simulink library "ddm"  (R2021b)
settings: Solver=VariableStepAuto  StartTime=0.0  StopTime=10.0  RelTol=1e-3
undefined symbols (not defined in the file): ADDM_FrTMTqDev_X_Nm, ADDM_RrTMTqDev_X_Nm, ENUM_ADASACCSTA_ERROR, ENUM_ADASACCSTA_OFF, ENUM_ADASACCSTA_STANDBY, ENUM_ALLOWMOV_ALLOWREADY, ENUM_APS, ENUM_BRKSTA_ERROR, ENUM_BRKSTA_OFF, ENUM_BRKSTA_ON, ENUM_BRKSW_INVALID, ENUM_BRKSW_OFF, ENUM_BRKSW_ON, ENUM_CHGPREACTERRSTA_OBCPRE, ENUM_DCDCFAULTSTA_ANYFAULTLV1, ENUM_DCDCFAULTSTA_ANYFAULTLV2, ENUM_DRIVETRAIN_AWD, ENUM_DRIVETRAIN_FWD, ENUM_DRIVETRAIN_RWD, ENUM_EDUDRTSTA_NORMAL, ENUM_EPBERROR_FAILED, ENUM_EPBSTA_APPLIED, ENUM_EPBSTA_RELEASED, ENUM_ESCAPSSta_APSUNAVAILABLE, ENUM_GEARACTUALPOSN_INVALID, ENUM_GEARACTUALPOSN_P, ENUM_HVBATTREADYPRE_READY, ENUM_HWRESETSTA_HWRESETING, ENUM_MCUWARN_LV0, ENUM_MCUWARN_LV1, ENUM_MCUWARN_LV2, ENUM_MCUWARN_LV3, ENUM_MCUWARN_NOERROR, ENUM_OBCFAULTSTA_ANYFAULT, ENUM_PAS_R2F2, ENUM_PDFAULT_BATTPDFAIL, ENUM_PDFAULT_DCDCDISABLE, ENUM_PDFAULT_MCUDISABLE, ENUM_PDFAULT_MCUDISCHRG, ENUM_POWERSTA_OFF, ENUM_POWERSTA_ON, ENUM_POWERSTA_READY, ENUM_POWERSTA_STANDBY, ENUM_PRESSINDI_LOW, ENUM_PUFAULT_BATTUPFAIL, ENUM_PUFAULT_DCDCENABLEFAIL, ENUM_PUFAULT_PRECHRGCHKFAIL, ENUM_PUFAULT_SAFETYCHKFAIL, ENUM_PWRSTASW_OFF, ENUM_PWRSTASW_OFFA, ENUM_PWRSTASW_OFFCHVCHRG, ENUM_PWRSTASW_OFFCLVCHRG, ENUM_PWRSTASW_ON, ENUM_PWRSTASW_ONHVCHRG, ENUM_PWRSTASW_READY, ENUM_PWRSTASW_STANDBY, ENUM_RAPSErrWarnSta_NORMAL, ENUM_RAPSErrWarnSta_RAPSERRLV1, ENUM_SHIFTCOMMAND_P, ENUM_SHIFTERERRSTA_PBUTTONFAILURE ... (+471)
libraries: hcu_lib x540, simulink x3
(part 8 of 26)

== system ddm/DDM/DDM/APM/Subsystem5 ==
  USSSta_flg : Inport
  VPMM_SysPwrSta_enum : Inport  Port=2
  VAPM_SNSRLayout_enum : Inport  Port=3
  Constant1 : Constant  Value=ENUM_PWRSTASW_READY
  Constant17 : Constant  Value=ENUM_PWRSTASW_READY
  Constant2 : Constant  Value=ENUM_PWRSTASW_ON
  Constant25 : Constant  Value=FALSE
  Constant3 : Constant  Value=ENUM_PWRSTASW_ON
  Constant4 : Constant  Value=ENUM_APS
  Constant5 : Constant  Value=ENUM_PAS_R2F2
  Equal{1..6} (6 alike) : RelationalOperator  Operator===  OutDataTypeStr=boolean  RndMeth=Simplest
  Logical Operator1 : Logic  Operator=NOT  AllPortsSameDT=off  OutDataTypeStr=boolean
  Logical Operator13 : Logic  Operator=OR  AllPortsSameDT=off  OutDataTypeStr=boolean
  Logical Operator2 : Logic  AllPortsSameDT=off  OutDataTypeStr=boolean
  Logical Operator3 : Logic  Operator=OR  AllPortsSameDT=off  OutDataTypeStr=boolean
  Logical Operator4 : Logic  AllPortsSameDT=off  OutDataTypeStr=boolean
  Logical Operator5 : Logic  Operator=OR  AllPortsSameDT=off  OutDataTypeStr=boolean
  Switch2 : Switch  Criteria=u2 ~= 0
  Pass_flg : Outport
  CFS_flg : Outport  Port=2
  wires:
  VPMM_SysPwrSta_enum/1 -> [VPMM_SysPwrSta_enum]
  Logical Operator4/1 -> CFS_flg/1
  Switch2/1 -> Logical Operator4/1, Logical Operator1/1
  [VPMM_SysPwrSta_enum] -> Equal1/1
  Equal3/1 -> Logical Operator3/1
  Constant1/1 -> Equal1/2
  Constant2/1 -> Equal3/2
  Equal1/1 -> Logical Operator3/2
  [VPMM_SysPwrSta_enum] -> Equal3/1
  Logical Operator3/1 -> Logical Operator4/2
  Logical Operator2/1 -> Pass_flg/1
  Logical Operator1/1 -> Logical Operator2/2
  Logical Operator13/1 -> Logical Operator2/1
  [VPMM_SysPwrSta_enum] -> Equal6/1
  Equal2/1 -> Logical Operator13/2
  Constant3/1 -> Equal6/2
  Constant17/1 -> Equal2/2
  Equal6/1 -> Logical Operator13/1
  [VPMM_SysPwrSta_enum] -> Equal2/1
  USSSta_flg/1 -> Switch2/1
  Equal4/1 -> Logical Operator5/1
  Constant25/1 -> Switch2/3
  Constant4/1 -> Equal4/1
  VAPM_SNSRLayout_enum/1 -> Equal4/2, Equal5/1
  Logical Operator5/1 -> Switch2/2
  Equal5/1 -> Logical Operator5/2
  Constant5/1 -> Equal5/2

== system ddm/DDM/DDM/APM/Subsystem6 ==
  USSSta_flg : Inport
  VPMM_SysPwrSta_enum : Inport  Port=2
  VAPM_SNSRLayout_enum : Inport  Port=3
  Constant1 : Constant  Value=ENUM_PWRSTASW_READY
  Constant17 : Constant  Value=ENUM_PWRSTASW_READY
  Constant2 : Constant  Value=ENUM_PWRSTASW_ON
  Constant25 : Constant  Value=FALSE
  Constant3 : Constant  Value=ENUM_PWRSTASW_ON
  Constant4 : Constant  Value=ENUM_APS
  Constant5 : Constant  Value=ENUM_PAS_R2F2
  Equal{1..6} (6 alike) : RelationalOperator  Operator===  OutDataTypeStr=boolean  RndMeth=Simplest
  Logical Operator1 : Logic  Operator=NOT  AllPortsSameDT=off  OutDataTypeStr=boolean
  Logical Operator13 : Logic  Operator=OR  AllPortsSameDT=off  OutDataTypeStr=boolean
  Logical Operator2 : Logic  AllPortsSameDT=off  OutDataTypeStr=boolean
  Logical Operator3 : Logic  Operator=OR  AllPortsSameDT=off  OutDataTypeStr=boolean
  Logical Operator4 : Logic  AllPortsSameDT=off  OutDataTypeStr=boolean
  Logical Operator5 : Logic  Operator=OR  AllPortsSameDT=off  OutDataTypeStr=boolean
  Switch2 : Switch  Criteria=u2 ~= 0
  Pass_flg : Outport
  CFS_flg : Outport  Port=2
  wires:
  VPMM_SysPwrSta_enum/1 -> [VPMM_SysPwrSta_enum]
  Logical Operator4/1 -> CFS_flg/1
  Switch2/1 -> Logical Operator4/1, Logical Operator1/1
  [VPMM_SysPwrSta_enum] -> Equal1/1
  Equal3/1 -> Logical Operator3/1
  Constant1/1 -> Equal1/2
  Constant2/1 -> Equal3/2
  Equal1/1 -> Logical Operator3/2
  [VPMM_SysPwrSta_enum] -> Equal3/1
  Logical Operator3/1 -> Logical Operator4/2
  Logical Operator2/1 -> Pass_flg/1
  Logical Operator1/1 -> Logical Operator2/2
  Logical Operator13/1 -> Logical Operator2/1
  [VPMM_SysPwrSta_enum] -> Equal6/1
  Equal2/1 -> Logical Operator13/2
  Constant3/1 -> Equal6/2
  Constant17/1 -> Equal2/2
  Equal6/1 -> Logical Operator13/1
  [VPMM_SysPwrSta_enum] -> Equal2/1
  USSSta_flg/1 -> Switch2/1
  Equal4/1 -> Logical Operator5/1
  Constant25/1 -> Switch2/3
  Constant4/1 -> Equal4/1
  VAPM_SNSRLayout_enum/1 -> Equal4/2, Equal5/1
  Logical Operator5/1 -> Switch2/2
  Equal5/1 -> Logical Operator5/2
  Constant5/1 -> Equal5/2

== system ddm/DDM/DDM/APM/Subsystem7 ==
  USSSta_flg : Inport
  VPMM_SysPwrSta_enum : Inport  Port=2
  VAPM_SNSRLayout_enum : Inport  Port=3
  Constant1 : Constant  Value=ENUM_PWRSTASW_READY
  Constant17 : Constant  Value=ENUM_PWRSTASW_READY
  Constant2 : Constant  Value=ENUM_PWRSTASW_ON
  Constant25 : Constant  Value=FALSE
  Constant3 : Constant  Value=ENUM_PWRSTASW_ON
  Constant5 : Constant  Value=ENUM_APS
  Equal{1..3,5..6} (5 alike) : RelationalOperator  Operator===  OutDataTypeStr=boolean  RndMeth=Simplest
  Logical Operator1 : Logic  Operator=NOT  AllPortsSameDT=off  OutDataTypeStr=boolean
  Logical Operator13 : Logic  Operator=OR  AllPortsSameDT=off  OutDataTypeStr=boolean
  Logical Operator2 : Logic  AllPortsSameDT=off  OutDataTypeStr=boolean
  Logical Operator3 : Logic  Operator=OR  AllPortsSameDT=off  OutDataTypeStr=boolean
  Logical Operator4 : Logic  AllPortsSameDT=off  OutDataTypeStr=boolean
  Switch2 : Switch  Criteria=u2 ~= 0
  Pass_flg : Outport
  CFS_flg : Outport  Port=2
  wires:
  [VPMM_SysPwrSta_enum] -> Equal2/1
  Equal6/1 -> Logical Operator13/1
  Constant17/1 -> Equal2/2
  Constant3/1 -> Equal6/2
  Equal2/1 -> Logical Operator13/2
  [VPMM_SysPwrSta_enum] -> Equal6/1
  Logical Operator13/1 -> Logical Operator2/1
  Logical Operator1/1 -> Logical Operator2/2
  Logical Operator2/1 -> Pass_flg/1
  Logical Operator3/1 -> Logical Operator4/2
  [VPMM_SysPwrSta_enum] -> Equal3/1
  Equal1/1 -> Logical Operator3/2
  Constant2/1 -> Equal3/2
  Constant1/1 -> Equal1/2
  Equal3/1 -> Logical Operator3/1
  [VPMM_SysPwrSta_enum] -> Equal1/1
  Switch2/1 -> Logical Operator4/1, Logical Operator1/1
  Logical Operator4/1 -> CFS_flg/1
  VPMM_SysPwrSta_enum/1 -> [VPMM_SysPwrSta_enum]
  Constant5/1 -> Equal5/2
  VAPM_SNSRLayout_enum/1 -> Equal5/1
  Equal5/1 -> Switch2/2
  Constant25/1 -> Switch2/3
  USSSta_flg/1 -> Switch2/1

== system ddm/DDM/DDM/APM/Subsystem8 ==
  USSSta_flg : Inport
  VPMM_SysPwrSta_enum : Inport  Port=2
  VAPM_SNSRLayout_enum : Inport  Port=3
  Constant1 : Constant  Value=ENUM_PWRSTASW_READY
  Constant17 : Constant  Value=ENUM_PWRSTASW_READY
  Constant2 : Constant  Value=ENUM_PWRSTASW_ON
  Constant25 : Constant  Value=FALSE
  Constant3 : Constant  Value=ENUM_PWRSTASW_ON
  Constant5 : Constant  Value=ENUM_APS
  Equal{1..3,5..6} (5 alike) : RelationalOperator  Operator===  OutDataTypeStr=boolean  RndMeth=Simplest
  Logical Operator1 : Logic  Operator=NOT  AllPortsSameDT=off  OutDataTypeStr=boolean
  Logical Operator13 : Logic  Operator=OR  AllPortsSameDT=off  OutDataTypeStr=boolean
  Logical Operator2 : Logic  AllPortsSameDT=off  OutDataTypeStr=boolean
  Logical Operator3 : Logic  Operator=OR  AllPortsSameDT=off  OutDataTypeStr=boolean
  Logical Operator4 : Logic  AllPortsSameDT=off  OutDataTypeStr=boolean
  Switch2 : Switch  Criteria=u2 ~= 0
  Pass_flg : Outport
  CFS_flg : Outport  Port=2
  wires:
  [VPMM_SysPwrSta_enum] -> Equal2/1
  Equal6/1 -> Logical Operator13/1
  Constant17/1 -> Equal2/2
  Constant3/1 -> Equal6/2
  Equal2/1 -> Logical Operator13/2
  [VPMM_SysPwrSta_enum] -> Equal6/1
  Logical Operator13/1 -> Logical Operator2/1
  Logical Operator1/1 -> Logical Operator2/2
  Logical Operator2/1 -> Pass_flg/1
  Logical Operator3/1 -> Logical Operator4/2
  [VPMM_SysPwrSta_enum] -> Equal3/1
  Equal1/1 -> Logical Operator3/2
  Constant2/1 -> Equal3/2
  Constant1/1 -> Equal1/2
  Equal3/1 -> Logical Operator3/1
  [VPMM_SysPwrSta_enum] -> Equal1/1
  Switch2/1 -> Logical Operator4/1, Logical Operator1/1
  Logical Operator4/1 -> CFS_flg/1
  VPMM_SysPwrSta_enum/1 -> [VPMM_SysPwrSta_enum]
  Constant5/1 -> Equal5/2
  VAPM_SNSRLayout_enum/1 -> Equal5/1
  Equal5/1 -> Switch2/2
  Constant25/1 -> Switch2/3
  USSSta_flg/1 -> Switch2/1

== system ddm/DDM/DDM/APM/Subsystem9 ==
  USSSta_flg : Inport
  VPMM_SysPwrSta_enum : Inport  Port=2
  VAPM_SNSRLayout_enum : Inport  Port=3
  Constant1 : Constant  Value=ENUM_PWRSTASW_READY
  Constant17 : Constant  Value=ENUM_PWRSTASW_READY
  Constant2 : Constant  Value=ENUM_PWRSTASW_ON
  Constant25 : Constant  Value=FALSE
  Constant3 : Constant  Value=ENUM_PWRSTASW_ON
  Constant5 : Constant  Value=ENUM_APS
  Equal{1..3,5..6} (5 alike) : RelationalOperator  Operator===  OutDataTypeStr=boolean  RndMeth=Simplest
  Logical Operator1 : Logic  Operator=NOT  AllPortsSameDT=off  OutDataTypeStr=boolean
  Logical Operator13 : Logic  Operator=OR  AllPortsSameDT=off  OutDataTypeStr=boolean
  Logical Operator2 : Logic  AllPortsSameDT=off  OutDataTypeStr=boolean
  Logical Operator3 : Logic  Operator=OR  AllPortsSameDT=off  OutDataTypeStr=boolean
  Logical Operator4 : Logic  AllPortsSameDT=off  OutDataTypeStr=boolean
  Switch2 : Switch  Criteria=u2 ~= 0
  Pass_flg : Outport
  CFS_flg : Outport  Port=2
  wires:
  [VPMM_SysPwrSta_enum] -> Equal2/1
  Equal6/1 -> Logical Operator13/1
  Constant17/1 -> Equal2/2
  Constant3/1 -> Equal6/2
  Equal2/1 -> Logical Operator13/2
  [VPMM_SysPwrSta_enum] -> Equal6/1
  Logical Operator13/1 -> Logical Operator2/1
  Logical Operator1/1 -> Logical Operator2/2
  Logical Operator2/1 -> Pass_flg/1
  Logical Operator3/1 -> Logical Operator4/2
  [VPMM_SysPwrSta_enum] -> Equal3/1
  Equal1/1 -> Logical Operator3/2
  Constant2/1 -> Equal3/2
  Constant1/1 -> Equal1/2
  Equal3/1 -> Logical Operator3/1
  [VPMM_SysPwrSta_enum] -> Equal1/1
  Switch2/1 -> Logical Operator4/1, Logical Operator1/1
  Logical Operator4/1 -> CFS_flg/1
  VPMM_SysPwrSta_enum/1 -> [VPMM_SysPwrSta_enum]
  Constant5/1 -> Equal5/2
  VAPM_SNSRLayout_enum/1 -> Equal5/1
  Equal5/1 -> Switch2/2
  Constant25/1 -> Switch2/3
  USSSta_flg/1 -> Switch2/1

== system ddm/DDM/DDM/Enabled Subsystem/Subsystem ==
  KDDM_DTCClockerMax_cnt : Inport
  Trigger : TriggerPort  VariantControl=(inherit)  ZeroCross=off  PortDimensions=1
  Add : Sum
  Constant : Constant  Value=ZERO_INT
  Constant1 : Constant  Value=ONE_INT
  Data Type Conversion : DataTypeConversion  OutDataTypeStr=uint8
  Delay : Delay  DelayLength=1
  Relational Operator : RelationalOperator  OutDataTypeStr=boolean  RndMeth=Simplest
  Switch : Switch  Criteria=u2 > Threshold
  VDDM_DTCCounter_cnt : Outport
  wires:
  Data Type Conversion/1 -> [VDDM_DTCCounter_cnt]
  Switch/1 -> Data Type Conversion/1, Delay/1
  [VDDM_DTCCounter_cnt] -> VDDM_DTCCounter_cnt/1
  Constant1/1 -> Add/1
  Delay/1 -> Relational Operator/1, Add/2
  Add/1 -> Switch/3
  [KDDM_DTCClockerMax_cnt] -> Relational Operator/2
  Constant/1 -> Switch/1
  Relational Operator/1 -> Switch/2
  KDDM_DTCClockerMax_cnt/1 -> [KDDM_DTCClockerMax_cnt]

== system ddm/DDM/DDM/PMM/Brake switch signal abnormal1 ==
  task_time_s : Inport
  VPMM_PowerSta_enum : Inport  Port=2
  VINP_BrakeSWGPIO_flg : Inport  Port=3
  VINP_BrakeLampSW_flg : Inport  Port=4
  VINP_DrStdAErrSta_enum : Inport  Port=5
  VINP_BrkSWSta_flg : Inport  Port=6
  VINP_BrkPedalPosSta_enum : Inport  Port=7
  VINP_BrkPedalPos_pct : Inport  Port=8
  DTC_clear_request : Inport  Port=9
  VDDM_ClearZevDTCcmd_flg : Inport  Port=10
  VINP_BrkSwV_flg : Inport  Port=11
  VDDM_ESC5Err_flg : Inport  Port=12
  Brake switch signal abnormal : Subsystem
  Brake switch signal abnormal and no backup signal : Subsystem
  Constant : Constant  Value=TRUE
  Constant1 : Constant  Value=ENUM_BRKSTA_ERROR
  Constant2 : Constant  Value=ENUM_BRKSTA_ON
  Constant3 : Constant  Value=ENUM_BRKSTA_OFF
  Constant4 : Constant  Value=FALSE
  Constant5 : Constant  Value=ENUM_BRKSTA_ERROR
  Constant6 : Constant  Value=ENUM_BRKSTA_ON
  Constant7 : Constant  Value=ENUM_BRKSTA_OFF
  Constant8 : Constant  Value=KDDM_BrkPedalPos_pct
  Equal : RelationalOperator  Operator===  OutDataTypeStr=boolean  RndMeth=Simplest
  Equal1 : RelationalOperator  Operator===  OutDataTypeStr=boolean  RndMeth=Simplest
  Equal2 : RelationalOperator  OutDataTypeStr=boolean  RndMeth=Simplest
  Logical Operator : Logic  Operator=OR  Inputs=3  AllPortsSameDT=off  OutDataTypeStr=boolean
  Logical Operator1 : Logic  Operator=OR  AllPortsSameDT=off  OutDataTypeStr=boolean
  Subsystem : Subsystem
  Switch{,1..3} (4 alike) : Switch  Criteria=u2 > Threshold
  Terminator : Terminator
  VDDM_BrkSWErrDTC_raw32 : Outport
  VDDM_BrkSWNoBacDTC_raw32 : Outport  Port=2
  VDDM_BrakeSW_enum : Outport  Port=3
  VDDM_CANBrkSW2Sta_enum : Outport  Port=4
  VDDM_BrkPedalPosSta_enum : Outport  Port=5
  VDDM_BrkSWErrCFS_flg : Outport  Port=6
  VDDM_BrkSWNoBacCFS_flg : Outport  Port=7
  VDDM_VCUBrkSWSta_enum : Outport  Port=8
  VDDM_EDriveSysErrBrake_flg : Outport  Port=9
  wires:
  [VINP_BrkPedalPos_pct] -> Brake switch signal abnormal and no backup signal/5(VINP_BrkPedalPos_pct)
  [VINP_BrkPedalPos_pct] -> Brake switch signal abnormal/5(VINP_BrkPedalPos_pct)
  [VINP_BrkPedalPos_pct] -> Equal2/1
  VINP_BrkPedalPos_pct/1 -> [VINP_BrkPedalPos_pct]
  [VDDM_EDriveSysErrBrake_flg] -> VDDM_EDriveSysErrBrake_flg/1
  [VDDM_VCUBrkSWSta_enum] -> VDDM_VCUBrkSWSta_enum/1
  [VDDM_BrkSWNoBacCFS_flg] -> VDDM_BrkSWNoBacCFS_flg/1
  [VDDM_BrkSWErrCFS_flg] -> VDDM_BrkSWErrCFS_flg/1
  [task_time_s] -> Brake switch signal abnormal and no backup signal/1(task_time_s)
  [VPMM_PowerSta_enum] -> Brake switch signal abnormal and no backup signal/2(VPMM_PowerSta_enum)
  [VDDM_BrkSWNoBac_flg] -> Brake switch signal abnormal and no backup signal/3(BrkSWNoBac)
  [DTC_clear_request] -> Brake switch signal abnormal and no backup signal/4(DTC_clear_request)
  Brake switch signal abnormal and no backup signal/2(VDDM_BrkSWNoBacCFS_flg) -> [VDDM_EDriveSysErrBrake_flg], [VDDM_BrkSWNoBacCFS_flg]
  [VPMM_PowerSta_enum] -> Brake switch signal abnormal/2(VPMM_PowerSta_enum)
  Brake switch signal abnormal/2(VDDM_BrkSWErrCFS_flg) -> [VDDM_BrkSWErrCFS_flg]
  [task_time_s] -> Brake switch signal abnormal/1(task_time_s)
  VPMM_PowerSta_enum/1 -> [VPMM_PowerSta_enum]
  task_time_s/1 -> [task_time_s]
  VINP_DrStdAErrSta_enum/1 -> Equal/1
  Constant/1 -> Equal/2
  Equal/1 -> Logical Operator/3
  Switch1/1 -> Switch/3
  Logical Operator/1 -> Switch/2
  Constant1/1 -> Switch/1
  VINP_BrkSWSta_flg/1 -> Switch1/2
  Constant2/1 -> Switch1/1
  Constant3/1 -> Switch1/3
  Constant7/1 -> Switch3/3
  Constant6/1 -> Switch3/1
  Constant5/1 -> Switch2/1
  Logical Operator1/1 -> Switch2/2
  Switch3/1 -> Switch2/3
  Equal1/1 -> Logical Operator1/2
  Constant4/1 -> Equal1/2
  VINP_BrkPedalPosSta_enum/1 -> Equal1/1
  Constant8/1 -> Equal2/2
  Equal2/1 -> Switch3/2
  Brake switch signal abnormal/1(VDDM_BrkSWErrDTC_raw32) -> VDDM_BrkSWErrDTC_raw32/1
  Brake switch signal abnormal and no backup signal/1(VDDM_BrkSWNoBacDTC_raw32) -> VDDM_BrkSWNoBacDTC_raw32/1
  Switch/1 -> [VDDM_CANBrkSW2Sta_enum]  "VDDM_CANBrkSW2Sta_enum"
  Switch2/1 -> [VDDM_BrkPedalPosSta_enum]  "VDDM_BrkPedalPosSta_enum"
  [VDDM_BrkPedalPosSta_enum] -> VDDM_BrkPedalPosSta_enum/1
  [VDDM_CANBrkSW2Sta_enum] -> VDDM_CANBrkSW2Sta_enum/1
  [VDDM_BrakeSW_enum] -> VDDM_BrakeSW_enum/1
  DTC_clear_request/1 -> [DTC_clear_request]
  [VDDM_ClearZevDTCcmd_flg] -> Brake switch signal abnormal/4(DTC_clear_request)
  [VDDM_CANBrkSW2Sta_enum] -> Subsystem/1(VDDM_CANBSW2S_enum)
  [VDDM_BrkPedalPosSta_enum] -> Subsystem/4(BrkPedalPos_enum)
  VINP_BrakeSWGPIO_flg/1 -> Subsystem/2(BrakeSW)
  VINP_BrakeLampSW_flg/1 -> Subsystem/3(Brake_Stop_Lamp)
  Subsystem/1(BrkSWErr) -> [VDDM_BrkSWErr_flg]  "VDDM_BrkSWErr_flg"
  Subsystem/4(VDDM_BrakeSW_enum) -> [VDDM_VCUBrkSWSta_enum], [VDDM_BrakeSW_enum]  "VDDM_BrakeSW_enum"
  Subsystem/2(BrkSWNoBac) -> [VDDM_BrkSWNoBac_flg]  "VDDM_BrkSWNoBac_flg"
  Subsystem/3(BrkSWPass) -> Terminator/1  "VDDM_BrkSWPass_flg"
  [VDDM_BrkSWErr_flg] -> Brake switch signal abnormal/3(BrkSWErr)
  VINP_BrkSwV_flg/1 -> [VINP_BrkSwV_flg]
  [VINP_BrkSwV_flg] -> Logical Operator/2
  VDDM_ESC5Err_flg/1 -> [VDDM_ESC5Err_flg]
  [VDDM_ESC5Err_flg] -> Brake switch signal abnormal/6(VDDM_ESC5Err_flg)
  [VDDM_ESC5Err_flg] -> Logical Operator/1
  [VDDM_ESC5Err_flg] -> Logical Operator1/1
  [VDDM_ESC5Err_flg] -> Brake switch signal abnormal and no backup signal/6(VDDM_ESC5Err_flg)
  VDDM_ClearZevDTCcmd_flg/1 -> [VDDM_ClearZevDTCcmd_flg]

== system ddm/DDM/DDM/PMM/Comm err ==
  note: CAN3 BMS6
  note: CAN3 BMS1
  note: CAN3 CCU1
  note: CAN3 CCU2
  note: CAN1 ABM1
  task_time_s : Inport
  VPMM_PowerSta_enum : Inport  Port=2
  VPMM_PwrStaSW_enum : Inport  Port=3
  VDDM_C3BMS6RCChk_flg : Inport  Port=4
  VDDM_C3BMS6CSChk_flg : Inport  Port=5
  VDDM_C3BMS6LCChk_flg : Inport  Port=6
  VDDM_C3BMS1RCChk_flg : Inport  Port=7
  VDDM_C3BMS1CSChk_flg : Inport  Port=8
  VDDM_C3BMS1LCChk_flg : Inport  Port=9
  VDDM_C3CCU1RCChk_flg : Inport  Port=10
  VDDM_C3CCU1CSChk_flg : Inport  Port=11
  VDDM_C3CCU1LCChk_flg : Inport  Port=12
  VDDM_C3CCU2RCChk_flg : Inport  Port=13
  VDDM_C3CCU2CSChk_flg : Inport  Port=14
  VDDM_C3CCU2LCChk_flg : Inport  Port=15
  VDDM_C1ABM1RCChk_flg : Inport  Port=16
  VDDM_C1ABM1CSChk_flg : Inport  Port=17
  VDDM_C1ABM1LCChk_flg : Inport  Port=18
  No_CAN3_BUS_OFF : Inport  Port=19
  No_CAN1_BUS_OFF : Inport  Port=20
  DTC_clear_request : Inport  Port=21
  VDDM_ClearZevDTCcmd_flg : Inport  Port=22
  VPMM_HWResetSta_enum : Inport  Port=23
  OR : Logic  Operator=OR  Inputs=3  AllPortsSameDT=off  OutDataTypeStr=boolean
  OR2 : Logic  Operator=OR  Inputs=3  AllPortsSameDT=off  OutDataTypeStr=boolean
  OR3 : Logic  Operator=OR  Inputs=3  AllPortsSameDT=off  OutDataTypeStr=boolean
  The CAN signal between VCU and ABM1 is discontinuous : Subsystem
  The CAN signal between VCU and ABM1 is incomplete : Subsystem
  The CAN signal between VCU and BMS1 is discontinuous : Subsystem
  The CAN signal between VCU and BMS1 is incomplete : Subsystem
  The CAN signal between VCU and BMS6 is discontinuous1 : Subsystem
  The CAN signal between VCU and BMS6 is incomplete1 : Subsystem
  The CAN signal between VCU and CCU1 is discontinuous : Subsystem
  The CAN signal between VCU and CCU1 is incomplete : Subsystem
  The CAN signal between VCU and CCU2 is discontinuous : Subsystem
  The CAN signal between VCU and CCU2 is incomplete : Subsystem
  VCU lost communication with ABM1 : Subsystem
  VCU lost communication with BMS1 : Subsystem
  VCU lost communication with BMS6 : Subsystem
  VCU lost communication with CCU1 : Subsystem
  VCU lost communication with CCU2 : Subsystem
  VDDM_C3BMS6RCDTC_raw32 : Outport
  VDDM_C3BMS6CSDTC_raw32 : Outport  Port=2
  VDDM_C3BMS6LCDTC_raw32 : Outport  Port=3
  VDDM_C3BMS1RCDTC_raw32 : Outport  Port=4
  VDDM_C3BMS1CSDTC_raw32 : Outport  Port=5
  VDDM_C3BMS1LCDTC_raw32 : Outport  Port=6
  VDDM_C3CCU1RCDTC_raw32 : Outport  Port=7
  VDDM_C3CCU1CSDTC_raw32 : Outport  Port=8
  VDDM_C3CCU1LCDTC_raw32 : Outport  Port=9
  VDDM_C3CCU2RCDTC_raw32 : Outport  Port=10
  VDDM_C3CCU2CSDTC_raw32 : Outport  Port=11
  VDDM_C3CCU2LCDTC_raw32 : Outport  Port=12
  VDDM_C1ABM1RCDTC_raw32 : Outport  Port=13
  VDDM_C1ABM1CSDTC_raw32 : Outport  Port=14
  VDDM_C1ABM1LCDTC_raw32 : Outport  Port=15
  VDDM_C3BMS6RCCFS_flg : Outport  Port=16
  VDDM_C3BMS6CSCFS_flg : Outport  Port=17
  VDDM_C3BMS6LCCFS_flg : Outport  Port=18
  VDDM_C3BMS1RCCFS_flg : Outport  Port=19
  VDDM_C3BMS1CSCFS_flg : Outport  Port=20
  VDDM_C3BMS1LCCFS_flg : Outport  Port=21
  VDDM_C3CCU1RCCFS_flg : Outport  Port=22
  VDDM_C3CCU1CSCFS_flg : Outport  Port=23
  VDDM_C3CCU1LCCFS_flg : Outport  Port=24
  VDDM_C3CCU2RCCFS_flg : Outport  Port=25
  VDDM_C3CCU2CSCFS_flg : Outport  Port=26
  VDDM_C3CCU2LCCFS_flg : Outport  Port=27
  VDDM_C1ABM1RCCFS_flg : Outport  Port=28
  VDDM_C1ABM1CSCFS_flg : Outport  Port=29
  VDDM_C1ABM1LCCFS_flg : Outport  Port=30
  VDDM_EDriveSysErrABMCAN_flg : Outport  Port=31
  VDDM_EDriveSysErrCCU1CAN_flg : Outport  Port=32
  VDDM_EDriveSysErrCCU2CAN_flg : Outport  Port=33
  wires:
  The CAN signal between VCU and CCU2 is discontinuous/2(VDDM_C3CCU2RCCFS_flg) -> [VDDM_C3CCU2RCCFS_flg], VDDM_C3CCU2RCCFS_flg/1
  The CAN signal between VCU and CCU2 is incomplete/2(VDDM_C3CCU2CSCFS_flg) -> [VDDM_C3CCU2CSCFS_flg], VDDM_C3CCU2CSCFS_flg/1
  The CAN signal between VCU and BMS6 is discontinuous1/2(VDDM_C3BMS6RCCFS_flg) -> VDDM_C3BMS6RCCFS_flg/1
  The CAN signal between VCU and BMS6 is incomplete1/2(VDDM_C3BMS6CSCFS_flg) -> VDDM_C3BMS6CSCFS_flg/1
  The CAN signal between VCU and CCU1 is discontinuous/1(VDDM_C3CCU1RCDTC_raw32) -> VDDM_C3CCU1RCDTC_raw32/1
  VCU lost communication with BMS6/1(VDDM_C3BMS6LCDTC_raw32) -> VDDM_C3BMS6LCDTC_raw32/1
  VCU lost communication with ABM1/1(VDDM_C1ABM1LCDTC_raw32) -> VDDM_C1ABM1LCDTC_raw32/1
  The CAN signal between VCU and ABM1 is incomplete/1(VDDM_C1ABM1CSDTC_raw32) -> VDDM_C1ABM1CSDTC_raw32/1
  The CAN signal between VCU and ABM1 is discontinuous/1(VDDM_C1ABM1RCDTC_raw32) -> VDDM_C1ABM1RCDTC_raw32/1
  VCU lost communication with CCU2/1(VDDM_C3CCU2LCDTC_raw32) -> VDDM_C3CCU2LCDTC_raw32/1
  The CAN signal between VCU and CCU2 is incomplete/1(VDDM_C3CCU2CSDTC_raw32) -> VDDM_C3CCU2CSDTC_raw32/1
  The CAN signal between VCU and CCU2 is discontinuous/1(VDDM_C3CCU2RCDTC_raw32) -> VDDM_C3CCU2RCDTC_raw32/1
  VCU lost communication with CCU1/1(VDDM_C3CCU1LCDTC_raw32) -> VDDM_C3CCU1LCDTC_raw32/1
  The CAN signal between VCU and CCU1 is incomplete/1(VDDM_C3CCU1CSDTC_raw32) -> VDDM_C3CCU1CSDTC_raw32/1
  VCU lost communication with BMS1/1(VDDM_C3BMS1LCDTC_raw32) -> VDDM_C3BMS1LCDTC_raw32/1
  The CAN signal between VCU and BMS1 is incomplete/1(VDDM_C3BMS1CSDTC_raw32) -> VDDM_C3BMS1CSDTC_raw32/1
  The CAN signal between VCU and BMS1 is discontinuous/1(VDDM_C3BMS1RCDTC_raw32) -> VDDM_C3BMS1RCDTC_raw32/1
  The CAN signal between VCU and BMS6 is incomplete1/1(VDDM_C3BMS6CSDTC_raw32) -> VDDM_C3BMS6CSDTC_raw32/1
  The CAN signal between VCU and BMS6 is discontinuous1/1(VDDM_C3BMS6RCDTC_raw32) -> VDDM_C3BMS6RCDTC_raw32/1
  DTC_clear_request/1 -> [DTC_clear_request]
  No_CAN1_BUS_OFF/1 -> [No_CAN1_BUS_OFF]
  No_CAN3_BUS_OFF/1 -> [No_CAN3_BUS_OFF]
  OR/1 -> VDDM_EDriveSysErrABMCAN_flg/1
  [VDDM_EDriveSysErrABMLC_flg] -> OR/3
  [VDDM_EDriveSysErrABMRC_flg] -> OR/1
  [VDDM_EDriveSysErrABMCS_flg] -> OR/2
  VCU lost communication with ABM1/3(LC_EDriveSysErr_VCUErr_flg) -> [VDDM_EDriveSysErrABMLC_flg]
  [DTC_clear_request] -> VCU lost communication with ABM1/6(DTC_clear_request)
  [No_CAN1_BUS_OFF] -> VCU lost communication with ABM1/5(No_CAN1_BUS_OFF)
  The CAN signal between VCU and ABM1 is incomplete/2(CS_EDriveSysErr_VCUErr_flg) -> [VDDM_EDriveSysErrABMCS_flg]
  The CAN signal between VCU and ABM1 is discontinuous/2(RC_EDriveSysErr_VCUErr_flg) -> [VDDM_EDriveSysErrABMRC_flg]
  [DTC_clear_request] -> The CAN signal between VCU and ABM1 is incomplete/7(DTC_clear_request)
  [No_CAN1_BUS_OFF] -> The CAN signal between VCU and ABM1 is incomplete/6(No_CAN1_BUS_OFF)
  [DTC_clear_request] -> The CAN signal between VCU and ABM1 is discontinuous/7(DTC_clear_request)
  [No_CAN1_BUS_OFF] -> The CAN signal between VCU and ABM1 is discontinuous/6(No_CAN1_BUS_OFF)
  [VDDM_ClearZevDTCcmd_flg] -> VCU lost communication with CCU1/6(DTC_clear_request)
  [No_CAN3_BUS_OFF] -> VCU lost communication with CCU1/5(No_CAN3_BUS_OFF)
  [VDDM_ClearZevDTCcmd_flg] -> VCU lost communication with BMS1/6(DTC_clear_request)
  [No_CAN3_BUS_OFF] -> VCU lost communication with BMS1/5(No_CAN3_BUS_OFF)
  [VDDM_ClearZevDTCcmd_flg] -> The CAN signal between VCU and BMS1 is incomplete/7(DTC_clear_request)
  [No_CAN3_BUS_OFF] -> The CAN signal between VCU and BMS1 is incomplete/6(No_CAN3_BUS_OFF)
  [VDDM_ClearZevDTCcmd_flg] -> The CAN signal between VCU and BMS1 is discontinuous/7(DTC_clear_request)
  [VDDM_ClearZevDTCcmd_flg] -> VCU lost communication with BMS6/6(DTC_clear_request)
  [VDDM_C3BMS6LCCFS_flg] -> The CAN signal between VCU and BMS6 is incomplete1/5(VDDM_C3BMS6LCCFS_flg)
  [VDDM_ClearZevDTCcmd_flg] -> The CAN signal between VCU and BMS6 is incomplete1/7(DTC_clear_request)
  VDDM_C3BMS6LCChk_flg/1 -> VCU lost communication with BMS6/4(VDDM_C3BMS6LCChk_flg)
  VDDM_C3BMS6CSChk_flg/1 -> The CAN signal between VCU and BMS6 is incomplete1/4(VDDM_C3BMS6CSChk_flg)
  task_time_s/1 -> [task_time_s]
  VPMM_PwrStaSW_enum/1 -> [VPMM_PwrStaSW_enum]
  VPMM_PowerSta_enum/1 -> [VPMM_PowerSta_enum]
  VDDM_C3CCU1CSChk_flg/1 -> The CAN signal between VCU and CCU1 is incomplete/4(VDDM_C3CCU1CSChk_flg)
  VDDM_C3BMS1CSChk_flg/1 -> The CAN signal between VCU and BMS1 is incomplete/4(VDDM_C3BMS1CSChk_flg)
  VDDM_C1ABM1CSChk_flg/1 -> The CAN signal between VCU and ABM1 is incomplete/4(VDDM_C1ABM1CSChk_flg)
  VDDM_C1ABM1RCChk_flg/1 -> The CAN signal between VCU and ABM1 is discontinuous/4(VDDM_C1ABM1RCChk_flg)
  VDDM_C3CCU1LCChk_flg/1 -> VCU lost communication with CCU1/4(VDDM_C3CCU1LCChk_flg)
  VDDM_C3BMS1RCChk_flg/1 -> The CAN signal between VCU and BMS1 is discontinuous/4(VDDM_C3BMS1RCChk_flg)
  [VPMM_PowerSta_enum] -> The CAN signal between VCU and ABM1 is discontinuous/2(VPMM_PowerSta_enum)
  [task_time_s] -> The CAN signal between VCU and ABM1 is discontinuous/1(task_time_s)
  [VDDM_C1ABM1LCCFS_flg] -> The CAN signal between VCU and ABM1 is incomplete/5(VDDM_C1ABM1LCCFS_flg)
  [VPMM_PowerSta_enum] -> The CAN signal between VCU and ABM1 is incomplete/2(VPMM_PowerSta_enum)
  [VPMM_PowerSta_enum] -> VCU lost communication with CCU2/2(VPMM_PowerSta_enum)
  VCU lost communication with BMS6/2(VDDM_C3BMS6LCCFS_flg) -> VDDM_C3BMS6LCCFS_flg/1, [VDDM_C3BMS6LCCFS_flg]
  [VPMM_PwrStaSW_enum] -> VCU lost communication with CCU1/3(VPMM_PwrStaSW_enum)
  [VPMM_PowerSta_enum] -> VCU lost communication with CCU1/2(VPMM_PowerSta_enum)
  [VPMM_PwrStaSW_enum] -> The CAN signal between VCU and CCU1 is incomplete/3(VPMM_PwrStaSW_enum)
  [task_time_s] -> The CAN signal between VCU and CCU1 is discontinuous/1(task_time_s)
  [VPMM_PowerSta_enum] -> The CAN signal between VCU and CCU1 is incomplete/2(VPMM_PowerSta_enum)
  VCU lost communication with CCU1/2(VDDM_C3CCU1LCCFS_flg) -> [VDDM_C3CCU1LCCFS_flg], VDDM_C3CCU1LCCFS_flg/1
  [task_time_s] -> VCU lost communication with BMS1/1(task_time_s)
  [VPMM_PowerSta_enum] -> VCU lost communication with BMS6/2(VPMM_PowerSta_enum)
  [VPMM_PwrStaSW_enum] -> The CAN signal between VCU and BMS1 is incomplete/3(VPMM_PwrStaSW_enum)
  [task_time_s] -> VCU lost communication with CCU1/1(task_time_s)
  [VDDM_C3BMS1LCCFS_flg] -> The CAN signal between VCU and BMS1 is incomplete/5(VDDM_C3BMS1LCCFS_flg)
  [VPMM_PowerSta_enum] -> The CAN signal between VCU and BMS1 is incomplete/2(VPMM_PowerSta_enum)
  VDDM_C3BMS1LCChk_flg/1 -> VCU lost communication with BMS1/4(VDDM_C3BMS1LCChk_flg)
  [task_time_s] -> The CAN signal between VCU and ABM1 is incomplete/1(task_time_s)
  [VPMM_PowerSta_enum] -> The CAN signal between VCU and BMS1 is discontinuous/2(VPMM_PowerSta_enum)
  [VPMM_PwrStaSW_enum] -> VCU lost communication with BMS1/3(VPMM_PwrStaSW_enum)
  [VPMM_PowerSta_enum] -> The CAN signal between VCU and BMS6 is incomplete1/2(VPMM_PowerSta_enum)
  [VPMM_PwrStaSW_enum] -> The CAN signal between VCU and BMS1 is discontinuous/3(VPMM_PwrStaSW_enum)
  [task_time_s] -> The CAN signal between VCU and BMS1 is discontinuous/1(task_time_s)
  [VPMM_PowerSta_enum] -> VCU lost communication with BMS1/2(VPMM_PowerSta_enum)
  VCU lost communication with BMS1/2(VDDM_C3BMS1LCCFS_flg) -> [VDDM_C3BMS1LCCFS_flg], VDDM_C3BMS1LCCFS_flg/1
  [task_time_s] -> The CAN signal between VCU and CCU1 is incomplete/1(task_time_s)
  [VDDM_C1ABM1LCCFS_flg] -> The CAN signal between VCU and ABM1 is discontinuous/5(VDDM_C1ABM1LCCFS_flg)
  [task_time_s] -> The CAN signal between VCU and BMS6 is incomplete1/1(task_time_s)
  VDDM_C1ABM1LCChk_flg/1 -> VCU lost communication with ABM1/4(VDDM_C1ABM1LCChk_flg)
  [VPMM_PwrStaSW_enum] -> The CAN signal between VCU and ABM1 is incomplete/3(VPMM_PwrStaSW_enum)
  VCU lost communication with ABM1/2(VDDM_C1ABM1LCCFS_flg) -> [VDDM_C1ABM1LCCFS_flg], VDDM_C1ABM1LCCFS_flg/1
  [task_time_s] -> VCU lost communication with CCU2/1(task_time_s)
  [VPMM_PwrStaSW_enum] -> The CAN signal between VCU and ABM1 is discontinuous/3(VPMM_PwrStaSW_enum)
  [VPMM_PowerSta_enum] -> VCU lost communication with ABM1/2(VPMM_PowerSta_enum)
  [VPMM_PwrStaSW_enum] -> VCU lost communication with BMS6/3(VPMM_PwrStaSW_enum)
  [task_time_s] -> The CAN signal between VCU and BMS1 is incomplete/1(task_time_s)
  [task_time_s] -> VCU lost communication with ABM1/1(task_time_s)
  VCU lost communication with CCU2/2(VDDM_C3CCU2LCCFS_flg) -> VDDM_C3CCU2LCCFS_flg/1, [VDDM_C3CCU2LCCFS_flg]
  [VPMM_PwrStaSW_enum] -> VCU lost communication with ABM1/3(VPMM_PwrStaSW_enum)
  [task_time_s] -> The CAN signal between VCU and BMS6 is discontinuous1/1(task_time_s)
  [task_time_s] -> The CAN signal between VCU and CCU2 is discontinuous/1(task_time_s)
  [task_time_s] -> VCU lost communication with BMS6/1(task_time_s)
  [VPMM_PwrStaSW_enum] -> The CAN signal between VCU and BMS6 is incomplete1/3(VPMM_PwrStaSW_enum)
  The CAN signal between VCU and BMS1 is discontinuous/2(VDDM_C3BMS1RCCFS_flg) -> VDDM_C3BMS1RCCFS_flg/1
  The CAN signal between VCU and BMS1 is incomplete/2(VDDM_C3BMS1CSCFS_flg) -> VDDM_C3BMS1CSCFS_flg/1
  The CAN signal between VCU and CCU1 is discontinuous/2(VDDM_C3CCU1RCCFS_flg) -> [VDDM_C3CCU1RCCFS_flg], VDDM_C3CCU1RCCFS_flg/1
  The CAN signal between VCU and CCU1 is incomplete/2(VDDM_C3CCU1CSCFS_flg) -> [VDDM_C3CCU1CSCFS_flg], VDDM_C3CCU1CSCFS_flg/1
  The CAN signal between VCU and ABM1 is discontinuous/3(VDDM_C1ABM1RCCFS_flg) -> VDDM_C1ABM1RCCFS_flg/1
  The CAN signal between VCU and ABM1 is incomplete/3(VDDM_C1ABM1CSCFS_flg) -> VDDM_C1ABM1CSCFS_flg/1
  VDDM_ClearZevDTCcmd_flg/1 -> [VDDM_ClearZevDTCcmd_flg]
  VPMM_HWResetSta_enum/1 -> [VPMM_HWResetSta_enum]
  [No_CAN3_BUS_OFF] -> VCU lost communication with BMS6/5(No_CAN3_BUS_OFF)
  [VPMM_HWResetSta_enum] -> VCU lost communication with BMS6/7(VPMM_HWResetSta_enum)
  [No_CAN3_BUS_OFF] -> The CAN signal between VCU and BMS6 is incomplete1/6(No_CAN3_BUS_OFF)
  [VPMM_HWResetSta_enum] -> The CAN signal between VCU and BMS6 is incomplete1/8(VPMM_HWResetSta_enum)
  [VPMM_PowerSta_enum] -> The CAN signal between VCU and BMS6 is discontinuous1/2(VPMM_PowerSta_enum)
  [VDDM_C3BMS6LCCFS_flg] -> The CAN signal between VCU and BMS6 is discontinuous1/5(VDDM_C3BMS6LCCFS_flg)
  [No_CAN3_BUS_OFF] -> The CAN signal between VCU and BMS6 is discontinuous1/6(No_CAN3_BUS_OFF)
  [VDDM_ClearZevDTCcmd_flg] -> The CAN signal between VCU and BMS6 is discontinuous1/7(DTC_clear_request)
  [VPMM_HWResetSta_enum] -> The CAN signal between VCU and BMS6 is discontinuous1/8(VPMM_HWResetSta_enum)
  [VPMM_PwrStaSW_enum] -> The CAN signal between VCU and BMS6 is discontinuous1/3(VPMM_PwrStaSW_enum)
  VDDM_C3BMS6RCChk_flg/1 -> The CAN signal between VCU and BMS6 is discontinuous1/4(VDDM_C3BMS6RCChk_flg)
  [VPMM_HWResetSta_enum] -> VCU lost communication with BMS1/7(VPMM_HWResetSta_enum)
  [VPMM_HWResetSta_enum] -> The CAN signal between VCU and BMS1 is incomplete/8(VPMM_HWResetSta_enum)
  [VDDM_C3BMS1LCCFS_flg] -> The CAN signal between VCU and BMS1 is discontinuous/5(VDDM_C3BMS1LCCFS_flg)
  [No_CAN3_BUS_OFF] -> The CAN signal between VCU and BMS1 is discontinuous/6(No_CAN3_BUS_OFF)
  [VPMM_HWResetSta_enum] -> The CAN signal between VCU and BMS1 is discontinuous/8(VPMM_HWResetSta_enum)
  [VPMM_HWResetSta_enum] -> VCU lost communication with CCU1/7(VPMM_HWResetSta_enum)
  [VDDM_C3CCU1LCCFS_flg] -> The CAN signal between VCU and CCU1 is incomplete/5(VDDM_C3CCU1LCCFS_flg)
  [No_CAN3_BUS_OFF] -> The CAN signal between VCU and CCU1 is incomplete/6(No_CAN3_BUS_OFF)
  [VDDM_ClearZevDTCcmd_flg] -> The CAN signal between VCU and CCU1 is incomplete/7(DTC_clear_request)
  [VPMM_HWResetSta_enum] -> The CAN signal between VCU and CCU1 is incomplete/8(VPMM_HWResetSta_enum)
  [VPMM_PowerSta_enum] -> The CAN signal between VCU and CCU1 is discontinuous/2(VPMM_PowerSta_enum)
  [VPMM_PwrStaSW_enum] -> The CAN signal between VCU and CCU1 is discontinuous/3(VPMM_PwrStaSW_enum)
  [VDDM_C3CCU1LCCFS_flg] -> The CAN signal between VCU and CCU1 is discontinuous/5(VDDM_C3CCU1LCCFS_flg)
  [No_CAN3_BUS_OFF] -> The CAN signal between VCU and CCU1 is discontinuous/6(No_CAN3_BUS_OFF)
  [VDDM_ClearZevDTCcmd_flg] -> The CAN signal between VCU and CCU1 is discontinuous/7(DTC_clear_request)
  VDDM_C3CCU1RCChk_flg/1 -> The CAN signal between VCU and CCU1 is discontinuous/4(VDDM_C3CCU1RCChk_flg)
  [VPMM_HWResetSta_enum] -> The CAN signal between VCU and CCU1 is discontinuous/8(VPMM_HWResetSta_enum)
  [VPMM_PwrStaSW_enum] -> VCU lost communication with CCU2/3(VPMM_PwrStaSW_enum)
  VDDM_C3CCU2LCChk_flg/1 -> VCU lost communication with CCU2/4(VDDM_C3CCU2LCChk_flg)
  [No_CAN3_BUS_OFF] -> VCU lost communication with CCU2/5(No_CAN3_BUS_OFF)
  [VDDM_ClearZevDTCcmd_flg] -> VCU lost communication with CCU2/6(DTC_clear_request)
  [VPMM_HWResetSta_enum] -> VCU lost communication with CCU2/7(VPMM_HWResetSta_enum)
  VDDM_C3CCU2CSChk_flg/1 -> The CAN signal between VCU and CCU2 is incomplete/4(VDDM_C3CCU2CSChk_flg)
  [VDDM_C3CCU2LCCFS_flg] -> The CAN signal between VCU and CCU2 is incomplete/5(VDDM_C3CCU2LCCFS_flg)
  [task_time_s] -> The CAN signal between VCU and CCU2 is incomplete/1(task_time_s)
  [VPMM_PowerSta_enum] -> The CAN signal between VCU and CCU2 is incomplete/2(VPMM_PowerSta_enum)
  [VPMM_PwrStaSW_enum] -> The CAN signal between VCU and CCU2 is incomplete/3(VPMM_PwrStaSW_enum)
  [No_CAN3_BUS_OFF] -> The CAN signal between VCU and CCU2 is incomplete/6(No_CAN3_BUS_OFF)
  [VDDM_ClearZevDTCcmd_flg] -> The CAN signal between VCU and CCU2 is incomplete/7(DTC_clear_request)
  [VPMM_HWResetSta_enum] -> The CAN signal between VCU and CCU2 is incomplete/8(VPMM_HWResetSta_enum)
  [VPMM_PowerSta_enum] -> The CAN signal between VCU and CCU2 is discontinuous/2(VPMM_PowerSta_enum)
  [VPMM_PwrStaSW_enum] -> The CAN signal between VCU and CCU2 is discontinuous/3(VPMM_PwrStaSW_enum)
  VDDM_C3CCU2RCChk_flg/1 -> The CAN signal between VCU and CCU2 is discontinuous/4(VDDM_C3CCU2RCChk_flg)
  [VDDM_C3CCU2LCCFS_flg] -> The CAN signal between VCU and CCU2 is discontinuous/5(VDDM_C3CCU2LCCFS_flg)
  [No_CAN3_BUS_OFF] -> The CAN signal between VCU and CCU2 is discontinuous/6(No_CAN3_BUS_OFF)
  [VDDM_ClearZevDTCcmd_flg] -> The CAN signal between VCU and CCU2 is discontinuous/7(DTC_clear_request)
  [VPMM_HWResetSta_enum] -> The CAN signal between VCU and CCU2 is discontinuous/8(VPMM_HWResetSta_enum)
  [VDDM_C3CCU2CSCFS_flg] -> OR3/3
  [VDDM_C3CCU2LCCFS_flg] -> OR3/1
  [VDDM_C3CCU1CSCFS_flg] -> OR2/3
  OR3/1 -> VDDM_EDriveSysErrCCU2CAN_flg/1
  OR2/1 -> VDDM_EDriveSysErrCCU1CAN_flg/1
  [VDDM_C3CCU2RCCFS_flg] -> OR3/2
  [VDDM_C3CCU1RCCFS_flg] -> OR2/2
  [VDDM_C3CCU1LCCFS_flg] -> OR2/1
